simulink model "Lowpass_Filter"  (R2025a)
settings: Solver=VariableStepAuto  StartTime=0.0  StopTime=10.0  RelTol=1e-3
settings Model: Creator=Polarstern  LastModifiedBy=Polarstern

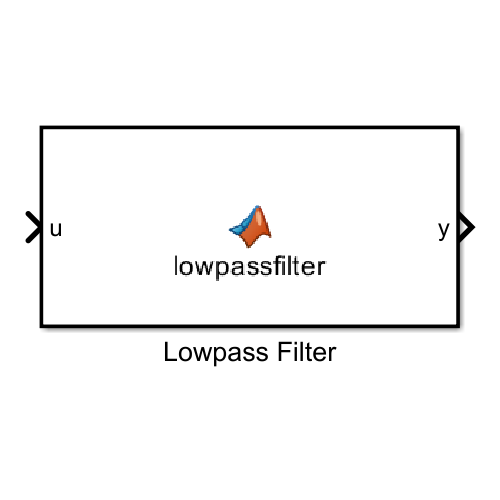
[thumbnail: Simulink's stored preview of the top-level diagram]
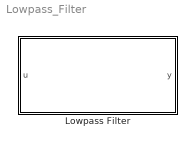
== system Lowpass_Filter ==
  Lowpass Filter : MATLAB Function  TreatAsAtomicUnit=on

== matlab function Lowpass_Filter/Lowpass Filter ==
  data: u input; y output
function y = lowpassfilter(u)
    %#codegen
    persistent z a b order initialized
    if isempty(initialized)
        initialized = true;
        load_data = load('lpf_params.mat');
        a = load_data.a;
        b = load_data.b;
        order = length(a) - 1;  % Detect order
        z = zeros(order, 1);  % States buffer
    end
    
    % Direct form II transposed
    temp = u;
    for i = 2:length(a)
        temp = temp - a(i) * z(i-1);
    end
    
    y = b(1) * temp;
    for i = 2:length(b)
        y = y + b(i) * z(i-1);
    end
    
    % Update states
    for i = order:-1:2
        z(i) = z(i-1);
    end
    z(1) = temp;

end
